simulink model "MPCdemo"  (R2023b)
settings: Solver=FixedStepAuto  StartTime=0.0  StopTime=10  FixedStep=0.01  RelTol=1e-3
settings Model: Creator=yxy  LastModifiedBy=17802
settings SolverCC: AlgebraicLoopSolver=TrustRegion
settings DataIOCC: ReturnWorkspaceOutputs=off
settings OptimizationCC: BlockReduction=off  DefaultParameterBehavior=Inlined  BufferReuse=off  ZeroExternalMemoryAtStartup=off  ZeroInternalMemoryAtStartup=off
settings DebuggingCC: UnconnectedInputMsg=warning  UnconnectedOutputMsg=warning  UnconnectedLineMsg=warning  ArithmeticOperatorsInVariantConditions=warning
settings ModelReferenceCC: EnableRefExpFcnMdlSchedulingChecks=on
settings SFSimCC: CustomCodeUndefinedFunction=UseInterfaceOnly  SimTargetLang=C++
settings RTWCC: TargetLang=C++
settings GRTTargetCC: TargetLangStandard=C++03 (ISO)  CodeInterfacePackaging=C++ class

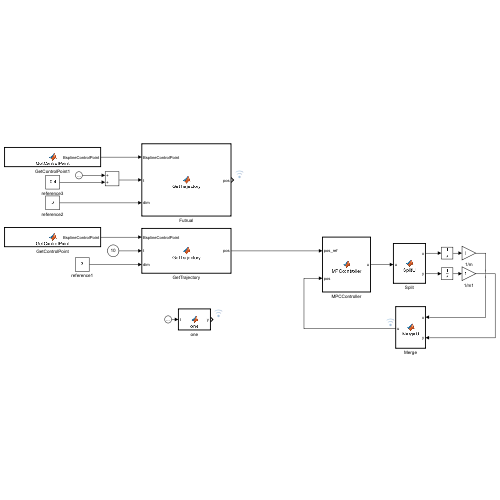
[thumbnail: Simulink's stored preview of the top-level diagram]
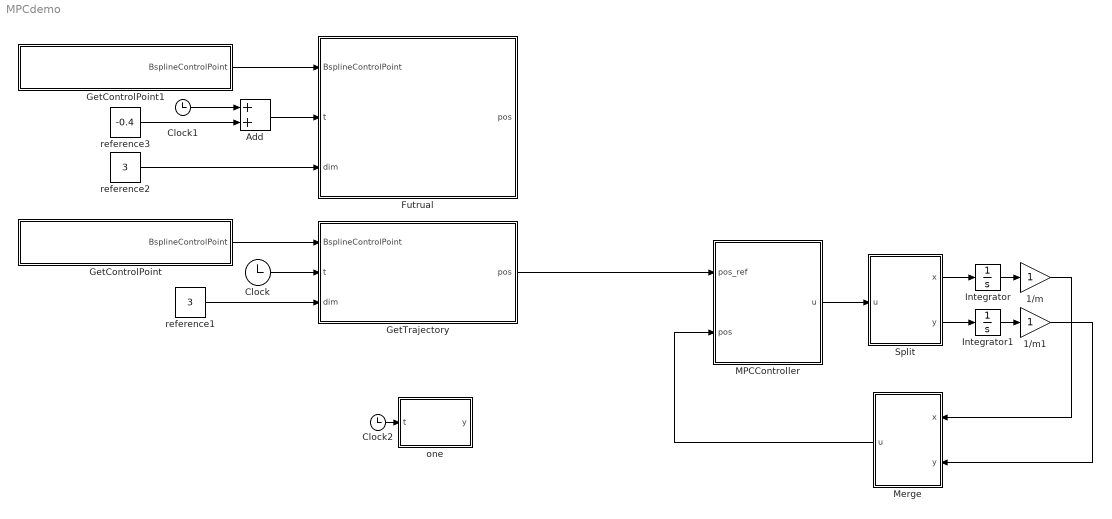
== system MPCdemo ==
  1/m : Gain
  1/m1 : Gain
  Add : Sum
  Clock : Clock
  Clock1 : Clock
  Clock2 : Clock
  Futrual : MATLAB Function  TreatAsAtomicUnit=on
  GetControlPoint : MATLAB Function  TreatAsAtomicUnit=on
  GetControlPoint1 : MATLAB Function  TreatAsAtomicUnit=on
  GetTrajectory : MATLAB Function  TreatAsAtomicUnit=on
  Integrator : Integrator  ContinuousStateAttributes='x'
  Integrator1 : Integrator  ContinuousStateAttributes='x'
  MPCController : MATLAB Function  TreatAsAtomicUnit=on
  Merge : MATLAB Function  TreatAsAtomicUnit=on
  Split : MATLAB Function  TreatAsAtomicUnit=on
  one : MATLAB Function  TreatAsAtomicUnit=on
  reference1 : Constant  Value=3
  reference2 : Constant  Value=3
  reference3 : Constant  Value=-0.4
  wires:
  Integrator/1 -> 1/m/1
  reference1/1 -> GetTrajectory/3(dim)
  GetControlPoint/1(BsplineControlPoint) -> GetTrajectory/1(BsplineControlPoint)
  Clock/1 -> GetTrajectory/2(t)
  MPCController/1(u) -> Split/1(u)
  Split/1(x) -> Integrator/1
  Split/2(y) -> Integrator1/1
  Integrator1/1 -> 1/m1/1
  1/m/1 -> Merge/1(x)
  1/m1/1 -> Merge/2(y)
  Merge/1(u) -> MPCController/2(pos)
  reference2/1 -> Futrual/3(dim)
  GetControlPoint1/1(BsplineControlPoint) -> Futrual/1(BsplineControlPoint)
  Add/1 -> Futrual/2(t)
  Clock1/1 -> Add/1
  reference3/1 -> Add/2
  Clock2/1 -> one/1(t)
  GetTrajectory/1(pos) -> MPCController/1(pos_ref)

== matlab function MPCdemo/GetTrajectory ==
  data: BsplineControlPoint input; t input; pos output; dim input
function pos = GetTrajectory(BsplineControlPoint,t,dim)
M_k = [1 / 6, 4 / 6, 1 / 6, 0;
    -3 / 6, 0, 3 / 6, 0;
    3 / 6, -6 / 6, 3 / 6, 0;
    -1 / 6, 3 / 6, -3 / 6, 1 / 6 ];
x = 0;
y = 0;
pos = [0 0]
t = min(t,size(BsplineControlPoint,1) - dim);
    u = t - floor(t);
    n = floor(t) + 1;
    pos(1) = [1,u,u*u,u*u*u]*M_k*BsplineControlPoint(n:n + 3,1);
    pos(2)  = [1,u,u*u,u*u*u]*M_k*BsplineControlPoint(n:n + 3,2);
end

== matlab function MPCdemo/Split ==
  data: x output; u input; y output
function [x,y] = SplitU(u)
x = u(1);
y = u(2);

== matlab function MPCdemo/GetControlPoint ==
  data: BsplineControlPoint output
function BsplineControlPoint = GetControlPoint
   
    BsplineControlPoint = [
        82.6672205185137	503.388274216037
        -3.83361025925683	594.305862891981
        82.6672205185137	503.388274216037
        137.367054362960	442.371791951226
        191.865226651865	385.590487038303
        232.772039029582	339.666259895562
        272.646617229806	332.944473379449
        295.441492051194	328.955846586641
        320.387414565418	328.832140273988
        352.608849687135	317.715592317407
        378.777186686044	303.505490456386
        408.682403568689	269.462445857051
        452.493199039199	236.244726115409
        461.275998627428	210.206751593442
        627.362000686286	196.396624203279
        461.275998627428	210.206751593442
        627.362000686286	196.396624203279
        ];

== matlab function MPCdemo/MPCController ==
  data: pos_ref input; u output; pos input
function u = MPCcontroller(pos_ref, pos)
%参数设置
T    = 0.01;           %控制周期10ms
p    = 40;            %控制时域（预测时域）
Q    = 10*eye(2*p);   %累计误差权重
W    = 0.0001*eye(2*p); %控制输出权重
umax = inf;           %控制量限制，即最大的力
Rk   = zeros(2*p,1);  %参考值序列
Rk(1:2:end) = pos_ref(1);    
Rk(2:2:end) = pos_ref(2);
%构建中间变量
xk    = [pos'];    %xk
A_    = [1 0;0 1];    %离散化预测模型参数A
B_    = [T 0;0 T];      %离散化预测模型参数B
psi   = zeros(2*p,2); %psi
for i=1:1:p
    psi(i*2-1:i*2,1:2)=A_^i;
end
theta = zeros(2*p,2*p); %theta
for i=1:1:p
    for j=1:1:i
        theta(i*2-1:i*2,j*2-1:j*2)=A_^(i-j)*B_;
    end
end
E = psi*xk-Rk;            %E
H = 2*(theta'*Q*theta+W); %H
f = (2*E'*Q*theta)';      %f
%优化求解
coder.extrinsic('quadprog');
Uk=quadprog(H,f,[],[],[],[],-umax,umax);
%返回控制量序列第一个值
u = [0,0];                %显示指定u的类型
u = [Uk(1),Uk(2)];

== matlab function MPCdemo/Merge ==
  data: u output; x input; y input
function u = MergeU(x,y)
u = [x,y];

== matlab function MPCdemo/GetControlPoint1 ==
  data: BsplineControlPoint output
function BsplineControlPoint = GetControlPoint
   
    BsplineControlPoint = [
        82.6672205185137	503.388274216037
        -3.83361025925683	594.305862891981
        82.6672205185137	503.388274216037
        137.367054362960	442.371791951226
        191.865226651865	385.590487038303
        232.772039029582	339.666259895562
        272.646617229806	332.944473379449
        295.441492051194	328.955846586641
        320.387414565418	328.832140273988
        352.608849687135	317.715592317407
        378.777186686044	303.505490456386
        408.682403568689	269.462445857051
        452.493199039199	236.244726115409
        461.275998627428	210.206751593442
        627.362000686286	196.396624203279
        461.275998627428	210.206751593442
        627.362000686286	196.396624203279
        ];

== matlab function MPCdemo/Futrual ==
  data: BsplineControlPoint input; t input; pos output; dim input
function pos = GetTrajectory(BsplineControlPoint,t,dim)
M_k = [1 / 6, 4 / 6, 1 / 6, 0;
    -3 / 6, 0, 3 / 6, 0;
    3 / 6, -6 / 6, 3 / 6, 0;
    -1 / 6, 3 / 6, -3 / 6, 1 / 6 ];
x = 0;
y = 0;
pos = [0 0]
t = max(0,min(t,size(BsplineControlPoint,1) - dim));
    u = t - floor(t);
    n = floor(t) + 1;
    pos(1) = [1,u,u*u,u*u*u]*M_k*BsplineControlPoint(n:n + 3,1);
    pos(2)  = [1,u,u*u,u*u*u]*M_k*BsplineControlPoint(n:n + 3,2);
end

== matlab function MPCdemo/one ==
  data: y output; t input
function y = one(t)
    y = [t,10];
